simulink model "moment_simulate"  (R2018a)
settings: Solver=FixedStepAuto  StartTime=0.0  StopTime=1000  FixedStep=dt  RelTol=1e-3
values from neighbouring files (symbols this model uses):
  dt = 0.01    [ACA_init.m]    (also in INIT_LINEAR.m; INIT_NDI.m)
  M_des = [0 -0.00014935494329 0.005058193947 -0.0809844391777 -0.136458117274 -0.0586992261394 -0.0209682853789 -0.0135038270766 -0.00442932636663 -0.00326693709023 -0.00126245467592 -0.000877256793288 ... (300003 elements, 100001x3)]    [M_des.mat]
settings Model: Creator=Meng Chaoheng  LastModifiedBy=Meng Chaoheng

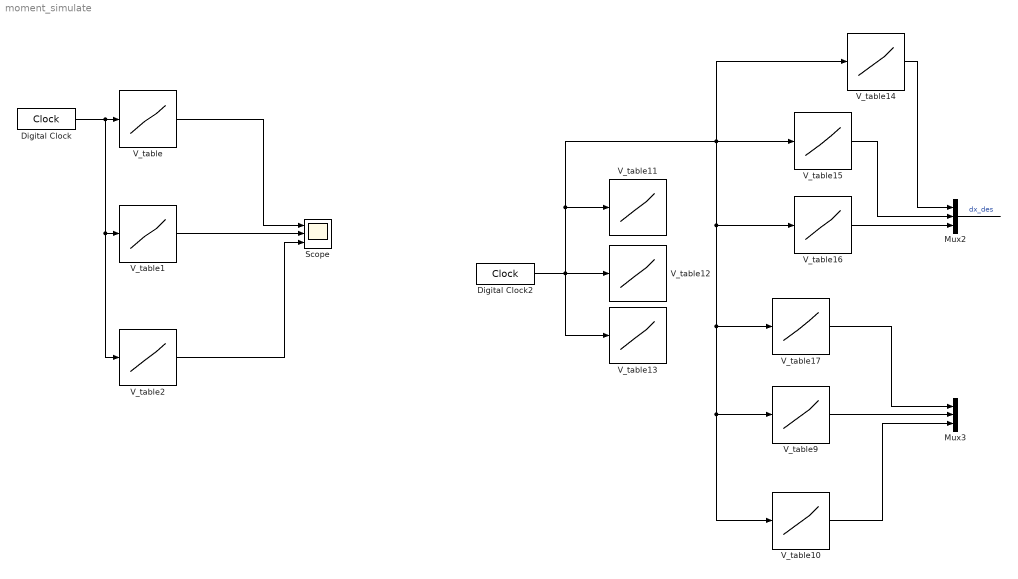
== system moment_simulate ==
  Digital Clock : DigitalClock  SampleTime=dt
  Digital Clock2 : DigitalClock  SampleTime=dt
  Mux2 : Mux  Inputs=3
  Mux3 : Mux  Inputs=3
  Scope : Scope  NumInputPorts=3
  V_table : Lookup  InputValues=t  Table=M_des(:,1)  LookUpMeth=Interpolation-Use End Values
  V_table1 : Lookup  InputValues=t  Table=M_des(:,2)  LookUpMeth=Interpolation-Use End Values
  V_table10 : Lookup  InputValues=t  Table=ones(length(t),1)*0  LookUpMeth=Interpolation-Use End Values
  V_table11 : Lookup  InputValues=t  Table=M_des(:,1)  LookUpMeth=Interpolation-Use End Values
  V_table12 : Lookup  InputValues=t  Table=M_des(:,2)  LookUpMeth=Interpolation-Use End Values
  V_table13 : Lookup  InputValues=t  Table=M_des(:,3)  LookUpMeth=Interpolation-Use End Values
  V_table14 : Lookup  InputValues=t  Table=0.0*sin(0.02*pi*t)  LookUpMeth=Interpolation-Use End Values
  V_table15 : Lookup  InputValues=t  Table=0.0*cos(0.02*pi*t)  LookUpMeth=Interpolation-Use End Values
  V_table16 : Lookup  InputValues=t  Table=0.0*cos(0.02*pi*t)  LookUpMeth=Interpolation-Use End Values
  V_table17 : Lookup  InputValues=t  Table=ones(length(t),1)*0  LookUpMeth=Interpolation-Use End Values
  V_table2 : Lookup  InputValues=t  Table=M_des(:,3)  LookUpMeth=Interpolation-Use End Values
  V_table9 : Lookup  InputValues=t  Table=ones(length(t),1)*0  LookUpMeth=Interpolation-Use End Values
  wires:
  Digital Clock/1 -> V_table1/1, V_table2/1, V_table/1
  V_table/1 -> Scope/1
  V_table1/1 -> Scope/2
  V_table2/1 -> Scope/3
  V_table17/1 -> Mux3/1
  V_table15/1 -> Mux2/2
  V_table16/1 -> Mux2/3
  V_table10/1 -> Mux3/3
  Digital Clock2/1 -> V_table14/1, V_table15/1, V_table16/1, V_table10/1, V_table9/1, V_table17/1, V_table11/1, V_table13/1, V_table12/1
  Mux2/1 -> ?  "dx_des"
  V_table14/1 -> Mux2/1
  V_table9/1 -> Mux3/2
